simulink model "Converter_simulink"  (R2026a)
settings: Solver=VariableStepAuto  StopTime=100
values from neighbouring files (symbols this model uses):
  C = 4*C_sc    (= 440)    [Simulink_Params.m]
  i_L0 = 0    [Simulink_Params.m]
  ki_pi = R/tau_i    (= 0.716283125018)    [Simulink_Params.m]
  kp_pi = L/tau_i    (= 0.00213422211966)    [Simulink_Params.m]
  L = d_max * v_l/ (f_sw * RR * I)    (= 2.03125e-05)    [Magnetics_Design.m]    (also in Simulink_Params.m = 2.8306e-05)
  R = 2 * R_on + R_l + R_esr/4    (= 0.0095)    [Simulink_Params.m]
  V_c0 = 2    [Simulink_Params.m]
  V_g = 24    [Simulink_Params.m]
libraries: simulink x4, slpidlib x1
settings Model: Creator=dhakk  LastModifiedBy=eganw

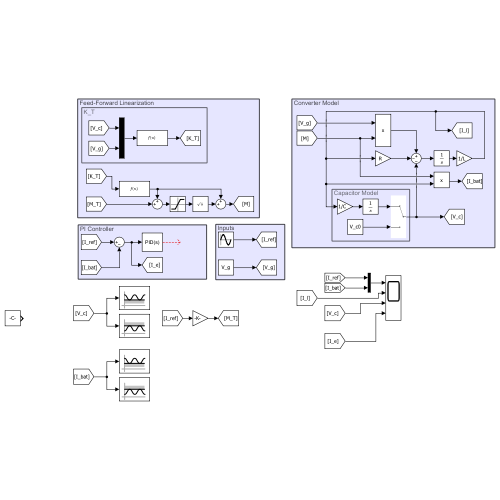
[thumbnail: Simulink's stored preview of the top-level diagram]
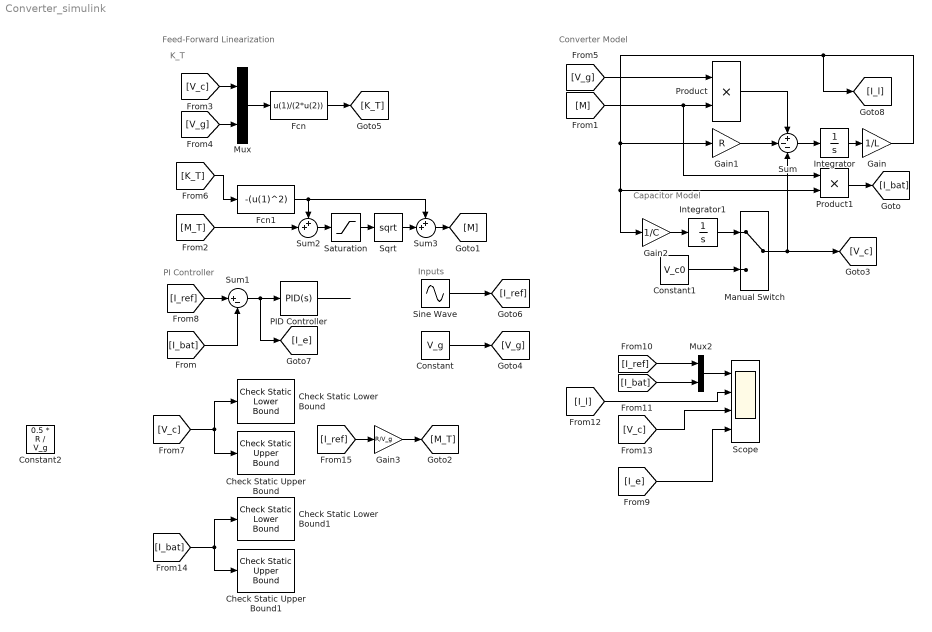
== system Converter_simulink ==
  note: Inputs
  note: PI Controller
  note: Capacitor Model
  note: Converter Model
  note: K_T
  note: Feed-Forward Linearization
  Check Static Lower Bound : simulink/Model Verification/Check Static  Lower Bound  Description=0 <= u  min=0  min_included=on  enabled=on  stopWhenAssertionFail=on  export=off  icon=graphic
  Check Static Lower Bound1 : simulink/Model Verification/Check Static  Lower Bound  Description=-30 <= u  min=-30  min_included=on  enabled=on  stopWhenAssertionFail=on  export=off  icon=graphic
  Check Static Upper Bound : simulink/Model Verification/Check Static  Upper Bound  Description=u <= 3  max=3  max_included=on  enabled=on  stopWhenAssertionFail=on  export=off  icon=graphic
  Check Static Upper Bound1 : simulink/Model Verification/Check Static  Upper Bound  Description=u <= 30  max=30  max_included=on  enabled=on  stopWhenAssertionFail=on  export=off  icon=graphic
  Constant : Constant  Value=V_g
  Constant1 : Constant  Value=V_c0
  Constant2 : Constant  Value=0.5 * R / V_g
  Fcn : Fcn  Expr=u(1)/(2*u(2))
  Fcn1 : Fcn  Expr=-(u(1)^2)
  Gain : Gain  Gain=1/L
  Gain1 : Gain  Gain=R
  Gain2 : Gain  Gain=1/C
  Gain3 : Gain  Gain=R/V_g
  Integrator : Integrator  InitialCondition=i_L0
  Integrator1 : Integrator  InitialCondition=V_c0
  Manual Switch : ManualSwitch
  Mux : Mux  Inputs=2
  Mux2 : Mux  Inputs=2
  PID Controller : slpidlib/PID Controller  Controller=PID  Form=Parallel  TimeDomain=Continuous-time  UseExternalTs=off  SampleTime=-1  IntegratorMethod=Forward Euler  FilterMethod=Forward Euler  ControllerParametersSource=internal  P=kp_pi  I=ki_pi  UseKiTs=off  D=0  UseExternalDerivativeSource=off  N=100  UseFilter=on  TunerSelectOption=Transfer Function Based (PID Tuner App)  InitialConditionSource=internal  InitialConditionForIntegrator=0  InitialConditionForFilter=0  DifferentiatorICPrevScaledInput=0  ExternalReset=none  TrackingMode=off  Kt=1  LimitOutput=off  SatLimitsSource=internal  UpperSaturationLimit=inf  LowerSaturationLimit=-inf  LinearizeAsGain=on  AntiWindupMode=none  Kb=1  LimitIntegrator=off  UpperIntegratorSaturationLimit=inf  LowerIntegratorSaturationLimit=-inf  POutMin=[]  POutMax=[]  IOutMin=[]  IOutMax=[]  DOutMin=[]  DOutMax=[]  NOutMin=[]  NOutMax=[]  SumOutMin=[]  SumOutMax=[]  SaturationOutMin=[]  SaturationOutMax=[]  PParamMin=[]  PParamMax=[]  IParamMin=[]  IParamMax=[]  DParamMin=[]  DParamMax=[]  NParamMin=[]  NParamMax=[]  KbParamMin=[]  KbParamMax=[]  KtParamMin=[]  KtParamMax=[]  KbOutMin=[]  KbOutMax=[]  KtOutMin=[]  KtOutMax=[]  IntegratorOutMin=[]  IntegratorOutMax=[]  FilterOutMin=[]  FilterOutMax=[]  SumI1OutMin=[]  SumI1OutMax=[]  SumI2OutMin=[]  SumI2OutMax=[]  SumI3OutMin=[]  SumI3OutMax=[]  SumI4OutMin=[]  SumI4OutMax=[]  SumDOutMin=[]  SumDOutMax=[]  DifferentiatorOutMin=[]  DifferentiatorOutMax=[]  FilterDiffOutCoefMin=[]  FilterDiffOutCoefMax=[]  ReciprocalOutMin=[]  ReciprocalOutMax=[]  SumDenOutMin=[]  SumDenOutMax=[]  SumNumOutMin=[]  SumNumOutMax=[]  DivideOutMin=[]  DivideOutMax=[]  UdiffTsProdOutMin=[]  UdiffTsProdOutMax=[]  NTsProdOutMin=[]  NTsProdOutMax=[]  UintegralTsProdOutMin=[]  UintegralTsProdOutMax=[]  UngainTsProdOutMin=[]  UngainTsProdOutMax=[]  ClampingZeroOutDataTypeStr=Inherit: Inherit via back propagation  ClampingZeroOutMin=[]  ClampingZeroOutMax=[]  FilterDenConstantOutDataTypeStr=Inherit: Inherit via back propagation  FilterDenConstantOutMin=[]  FilterDenConstantOutMax=[]  PCopyOutDataTypeStr=Inherit: Inherit via back propagation  PCopyOutMin=[]  PCopyOutMax=[]  NCopyOutDataTypeStr=Inherit: Inherit via back propagation  NCopyOutMin=[]  NCopyOutMax=[]  IntegratorContinuousStateAttributes=''  IntegratorStateMustResolveToSignalObject=off  IntegratorRTWStateStorageClass=Auto  FilterContinuousStateAttributes=''  FilterStateMustResolveToSignalObject=off  FilterRTWStateStorageClass=Auto  ParallelPVariant=InternalParameters  IdealPVariant=Disabled  IVariant=InternalParameters  DVariant=InternalParameters  IntegratorVariant=Continuous  SatVariant=Disabled  AWVariant=Passthrough  PCopyVariant=Disabled  TRVariant=Disabled  FdbkBlocksVariant=Forward  IdealPFdbkVariant=Disabled  SatFdbkVariant=Disabled  DerivativeFilterVariant=ContFilter  NVariant=InternalParameters  NCopyVariant=Disabled  FilterICVariant=InternalICsFilter  IntegratorICVariant=InternalICs  ExternalResetVariant=Disabled  TRSumVariant=Passthrough  SumFdbkVariant=Disabled  SumVariant=Sum_PID  TsampFilterVariant=InternalTs  TsampNgainVariant=Passthrough  TsampIntegralVariant=Disabled_SignalSpec  ExternalSaturationOutDataTypeStr=Inherit: Same as second input  DerivativeSourceVariant=ErrorSignal  PreIntVariant=InternalPreInt
  Product : Product
  Product1 : Product
  Saturation : Saturate  UpperLimit=inf  LowerLimit=0
  Scope : Scope  NumInputPorts=4
      settings: ActiveDisplayString=4  Title=Error Current  ActiveDisplayYMinimum=-483.51444469910524  ActiveDisplayYMaximum=473.64889102175135  YLabel=Current (Amps)
  Sine Wave : Sin  SampleTime=0
  Sqrt : Sqrt
  Sum : Sum  Inputs=+--
  Sum1 : Sum  Inputs=|+-
  Sum2 : Sum  Inputs=++|
  Sum3 : Sum  Inputs=++|
  wires:
  Integrator/1 -> Gain/1
  Product/1 -> Sum/1
  [V_g] -> Product/1
  [M] -> Product/2, Product1/1
  Gain1/1 -> Sum/2
  Sum/1 -> Integrator/1
  Gain/1 -> [I_l], Gain1/1, Product1/2, Gain2/1
  Manual Switch/1 -> Sum/3, [V_c]
  Gain2/1 -> Integrator1/1
  Product1/1 -> [I_bat]
  [I_ref] -> Sum1/1
  Sum1/1 -> [I_e], PID Controller/1
  [I_bat] -> Sum1/2
  PID Controller/1 -> ?
  Constant/1 -> [V_g]
  [V_g] -> Mux/2
  [V_c] -> Mux/1
  Mux/1 -> Fcn/1
  Fcn/1 -> [K_T]
  Fcn1/1 -> Sum3/1, Sum2/1
  [M_T] -> Sum2/2
  Sum2/1 -> Saturation/1
  Saturation/1 -> Sqrt/1
  [K_T] -> Fcn1/1
  Integrator1/1 -> Manual Switch/1
  Constant1/1 -> Manual Switch/2
  Sine Wave/1 -> [I_ref]
  [V_c] -> Check Static Upper Bound/1, Check Static Lower Bound/1
  [I_bat] -> Mux2/2
  [I_ref] -> Mux2/1
  Mux2/1 -> Scope/1
  [I_l] -> Scope/2
  [V_c] -> Scope/3
  [I_bat] -> Check Static Upper Bound1/1, Check Static Lower Bound1/1
  Sqrt/1 -> Sum3/2
  Sum3/1 -> [M]
  [I_e] -> Scope/4
  [I_ref] -> Gain3/1
  Gain3/1 -> [M_T]
